simulink model "pid_2dof_nonlinear_force"  (R2017a)
settings: Solver=ode45  StartTime=0.0  StopTime=10  RelTol=1e-3
undefined symbols (not defined in the file): f, g, GoalPos, l, m_p
libraries: simulink x2
settings Model: Creator=sansh  LastModifiedBy=rj2318

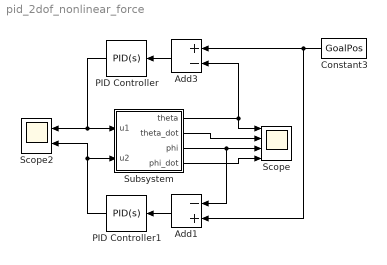
== system pid_2dof_nonlinear_force ==
  Add1 : Sum  Inputs=-+
  Add3 : Sum  Inputs=+-
  Constant3 : Constant  Value=GoalPos
  PID Controller : simulink/Continuous/PID Controller  Controller=PID  TimeDomain=Continuous-time  SampleTime=-1  IntegratorMethod=Forward Euler  FilterMethod=Forward Euler  Form=Parallel  UseFilter=on  ControllerParametersSource=internal  P=100  I=0.01  D=10  N=10  InitialConditionSource=internal  InitialConditionForIntegrator=0  InitialConditionForFilter=0  ExternalReset=none  LimitOutput=off  UpperSaturationLimit=inf  LowerSaturationLimit=-inf  LinearizeAsGain=on  AntiWindupMode=none  Kb=1  TrackingMode=off  Kt=1  PParamMin=[]  PParamMax=[]  IParamMin=[]  IParamMax=[]  DParamMin=[]  DParamMax=[]  NParamMin=[]  NParamMax=[]  KbParamMin=[]  KbParamMax=[]  KtParamMin=[]  KtParamMax=[]  POutMin=[]  POutMax=[]  IOutMin=[]  IOutMax=[]  DOutMin=[]  DOutMax=[]  NOutMin=[]  NOutMax=[]  KbOutMin=[]  KbOutMax=[]  KtOutMin=[]  KtOutMax=[]  IntegratorOutMin=[]  IntegratorOutMax=[]  FilterOutMin=[]  FilterOutMax=[]  SumOutMin=[]  SumOutMax=[]  SumI1OutMin=[]  SumI1OutMax=[]  SumI2OutMin=[]  SumI2OutMax=[]  SumI3OutMin=[]  SumI3OutMax=[]  SumDOutMin=[]  SumDOutMax=[]  SaturationOutMin=[]  SaturationOutMax=[]  IntegratorContinuousStateAttributes=''  IntegratorStateMustResolveToSignalObject=off  IntegratorRTWStateStorageClass=Auto  FilterContinuousStateAttributes=''  FilterStateMustResolveToSignalObject=off  FilterRTWStateStorageClass=Auto  DifferentiatorICPrevScaledInput=0  DifferentiatorOutMin=[]  DifferentiatorOutMax=[]
  PID Controller1 : simulink/Continuous/PID Controller  Controller=PID  TimeDomain=Continuous-time  SampleTime=-1  IntegratorMethod=Forward Euler  FilterMethod=Forward Euler  Form=Parallel  UseFilter=on  ControllerParametersSource=internal  P=100  I=0.01  D=10  N=10  InitialConditionSource=internal  InitialConditionForIntegrator=0  InitialConditionForFilter=0  ExternalReset=none  LimitOutput=off  UpperSaturationLimit=inf  LowerSaturationLimit=-inf  LinearizeAsGain=on  AntiWindupMode=none  Kb=1  TrackingMode=off  Kt=1  PParamMin=[]  PParamMax=[]  IParamMin=[]  IParamMax=[]  DParamMin=[]  DParamMax=[]  NParamMin=[]  NParamMax=[]  KbParamMin=[]  KbParamMax=[]  KtParamMin=[]  KtParamMax=[]  POutMin=[]  POutMax=[]  IOutMin=[]  IOutMax=[]  DOutMin=[]  DOutMax=[]  NOutMin=[]  NOutMax=[]  KbOutMin=[]  KbOutMax=[]  KtOutMin=[]  KtOutMax=[]  IntegratorOutMin=[]  IntegratorOutMax=[]  FilterOutMin=[]  FilterOutMax=[]  SumOutMin=[]  SumOutMax=[]  SumI1OutMin=[]  SumI1OutMax=[]  SumI2OutMin=[]  SumI2OutMax=[]  SumI3OutMin=[]  SumI3OutMax=[]  SumDOutMin=[]  SumDOutMax=[]  SaturationOutMin=[]  SaturationOutMax=[]  IntegratorContinuousStateAttributes=''  IntegratorStateMustResolveToSignalObject=off  IntegratorRTWStateStorageClass=Auto  FilterContinuousStateAttributes=''  FilterStateMustResolveToSignalObject=off  FilterRTWStateStorageClass=Auto  DifferentiatorICPrevScaledInput=0  DifferentiatorOutMin=[]  DifferentiatorOutMax=[]
  Scope : Scope  NumInputPorts=4
  Scope2 : Scope  NumInputPorts=2
  Subsystem : Subsystem
  wires:
  Subsystem/1(theta) -> Add3/2, Scope/1
  Subsystem/2(theta_dot) -> Scope/2
  Add3/1 -> PID Controller/1
  Subsystem/3(phi) -> Add1/1, Scope/3
  Constant3/1 -> Add3/1, Add1/2
  Subsystem/4(phi_dot) -> Scope/4
  Add1/1 -> PID Controller1/1
  PID Controller/1 -> Subsystem/1(u1), Scope2/1
  PID Controller1/1 -> Subsystem/2(u2), Scope2/2

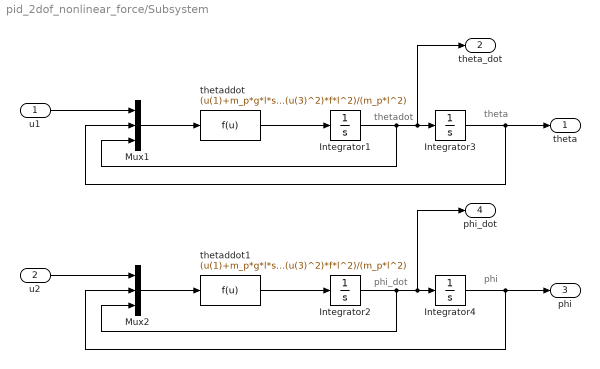
== system pid_2dof_nonlinear_force/Subsystem ==
  note: theta
  note: thetadot
  note: phi
  note: phi_dot
  u1 : Inport
  u2 : Inport  Port=2
  Integrator1 : Integrator  ContinuousStateAttributes='thetadot'
  Integrator2 : Integrator  ContinuousStateAttributes='thetadot'
  Integrator3 : Integrator  InitialCondition=0.1  ContinuousStateAttributes='theta'
  Integrator4 : Integrator  InitialCondition=0.1  ContinuousStateAttributes='theta'
  Mux1 : Mux  Inputs=3
  Mux2 : Mux  Inputs=3
  thetaddot : Fcn  Expr=(u(1)+m_p*g*l*sin(u(2))-(u(3)^2)*f*l^2)/(m_p*l^2)
  thetaddot1 : Fcn  Expr=(u(1)+m_p*g*l*sin(u(2))-(u(3)^2)*f*l^2)/(m_p*l^2)
  theta : Outport
  theta_dot : Outport  Port=2
  phi : Outport  Port=3
  phi_dot : Outport  Port=4
  wires:
  Mux1/1 -> thetaddot/1
  thetaddot/1 -> Integrator1/1
  Integrator1/1 -> Mux1/3, theta_dot/1, Integrator3/1
  Integrator3/1 -> Mux1/2, theta/1
  Integrator4/1 -> Mux2/2, phi/1
  thetaddot1/1 -> Integrator2/1
  Mux2/1 -> thetaddot1/1
  Integrator2/1 -> Mux2/3, phi_dot/1, Integrator4/1
  u1/1 -> Mux1/1
  u2/1 -> Mux2/1
